simulink model "Prueba_PID"  (R2015b)
settings: Solver=ode45  StartTime=0  StopTime=1000  FixedStep=0.001  RelTol=1e-3
libraries: simulink_extras x20, simulink x6, aerolibtransform2 x4, aerolibutil x4, aerolibobsolete x2, aerolibasang x2
(part 1 of 3)
settings Model: Creator=David  LastModifiedBy=Juan
settings SolverCC: InitialStep=AUTO
settings DataIOCC: SaveCompleteFinalSimState=on  SaveFormat=Array  SaveState=on  ReturnWorkspaceOutputsName=simout
settings DebuggingCC: AlgebraicLoopMsg=none  UnderspecifiedInitializationDetection=Classic  MergeDetectMultiDrivingBlocksExec=none  StateNameClashWarn=warning
settings HardwareCC: ProdBitPerPointer=32  ProdLargestAtomicFloat=None  ProdIntDivRoundTo=Undefined  ProdEndianess=Unspecified  ProdWordSize=32  ProdHWDeviceType=32-bit Generic
settings GRTTargetCC: GeneratePreprocessorConditionals=Disable all
settings ConfigComp: CovModelRefEnable=Off

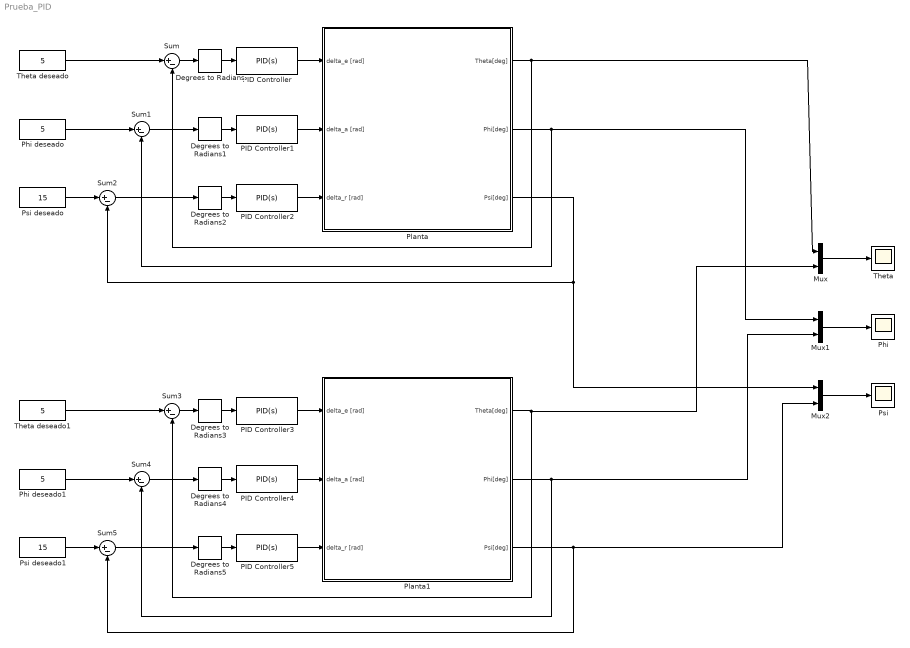
== system Prueba_PID ==
  Degrees to Radians{,1..5} (6 alike) : simulink_extras/Transformations/Degrees to Radians
  Mux : Mux  Inputs=2
  Mux1 : Mux  Inputs=2
  Mux2 : Mux  Inputs=2
  PID Controller : simulink/Continuous/PID Controller  Controller=PID  TimeDomain=Continuous-time  SampleTime=-1  IntegratorMethod=Forward Euler  FilterMethod=Forward Euler  Form=Parallel  UseFilter=on  ControllerParametersSource=internal  P=-1  I=-0.008  D=0.09  N=2  InitialConditionSource=internal  InitialConditionForIntegrator=0  InitialConditionForFilter=0  ExternalReset=none  LimitOutput=on  UpperSaturationLimit=0.062  LowerSaturationLimit=-0.062  LinearizeAsGain=on  AntiWindupMode=none  Kb=1  TrackingMode=off  Kt=1  PParamMin=[]  PParamMax=[]  IParamMin=[]  IParamMax=[]  DParamMin=[]  DParamMax=[]  NParamMin=[]  NParamMax=[]  KbParamMin=[]  KbParamMax=[]  KtParamMin=[]  KtParamMax=[]  POutMin=[]  POutMax=[]  IOutMin=[]  IOutMax=[]  DOutMin=[]  DOutMax=[]  NOutMin=[]  NOutMax=[]  KbOutMin=[]  KbOutMax=[]  KtOutMin=[]  KtOutMax=[]  IntegratorOutMin=[]  IntegratorOutMax=[]  FilterOutMin=[]  FilterOutMax=[]  SumOutMin=[]  SumOutMax=[]  SumI1OutMin=[]  SumI1OutMax=[]  SumI2OutMin=[]  SumI2OutMax=[]  SumI3OutMin=[]  SumI3OutMax=[]  SumDOutMin=[]  SumDOutMax=[]  SaturationOutMin=[]  SaturationOutMax=[]  IntegratorContinuousStateAttributes=''  IntegratorStateMustResolveToSignalObject=off  IntegratorRTWStateStorageClass=Auto  FilterContinuousStateAttributes=''  FilterStateMustResolveToSignalObject=off  FilterRTWStateStorageClass=Auto  DifferentiatorICPrevScaledInput=0  DifferentiatorOutMin=[]  DifferentiatorOutMax=[]
  PID Controller1 : simulink/Continuous/PID Controller  Controller=PID  TimeDomain=Continuous-time  SampleTime=-1  IntegratorMethod=Forward Euler  FilterMethod=Forward Euler  Form=Parallel  UseFilter=on  ControllerParametersSource=internal  P=0.09  I=0.001  D=2  N=2  InitialConditionSource=internal  InitialConditionForIntegrator=0  InitialConditionForFilter=0  ExternalReset=none  LimitOutput=on  UpperSaturationLimit=0.062  LowerSaturationLimit=-0.062  LinearizeAsGain=on  AntiWindupMode=none  Kb=1  TrackingMode=off  Kt=1  PParamMin=[]  PParamMax=[]  IParamMin=[]  IParamMax=[]  DParamMin=[]  DParamMax=[]  NParamMin=[]  NParamMax=[]  KbParamMin=[]  KbParamMax=[]  KtParamMin=[]  KtParamMax=[]  POutMin=[]  POutMax=[]  IOutMin=[]  IOutMax=[]  DOutMin=[]  DOutMax=[]  NOutMin=[]  NOutMax=[]  KbOutMin=[]  KbOutMax=[]  KtOutMin=[]  KtOutMax=[]  IntegratorOutMin=[]  IntegratorOutMax=[]  FilterOutMin=[]  FilterOutMax=[]  SumOutMin=[]  SumOutMax=[]  SumI1OutMin=[]  SumI1OutMax=[]  SumI2OutMin=[]  SumI2OutMax=[]  SumI3OutMin=[]  SumI3OutMax=[]  SumDOutMin=[]  SumDOutMax=[]  SaturationOutMin=[]  SaturationOutMax=[]  IntegratorContinuousStateAttributes=''  IntegratorStateMustResolveToSignalObject=off  IntegratorRTWStateStorageClass=Auto  FilterContinuousStateAttributes=''  FilterStateMustResolveToSignalObject=off  FilterRTWStateStorageClass=Auto  DifferentiatorICPrevScaledInput=0  DifferentiatorOutMin=[]  DifferentiatorOutMax=[]
  PID Controller2 : simulink/Continuous/PID Controller  Controller=PID  TimeDomain=Continuous-time  SampleTime=-1  IntegratorMethod=Forward Euler  FilterMethod=Forward Euler  Form=Parallel  UseFilter=on  ControllerParametersSource=internal  P=-0.5  I=-0.005  D=-0.01  N=2  InitialConditionSource=internal  InitialConditionForIntegrator=0  InitialConditionForFilter=0  ExternalReset=none  LimitOutput=on  UpperSaturationLimit=0.062  LowerSaturationLimit=-0.062  LinearizeAsGain=on  AntiWindupMode=none  Kb=1  TrackingMode=off  Kt=1  PParamMin=[]  PParamMax=[]  IParamMin=[]  IParamMax=[]  DParamMin=[]  DParamMax=[]  NParamMin=[]  NParamMax=[]  KbParamMin=[]  KbParamMax=[]  KtParamMin=[]  KtParamMax=[]  POutMin=[]  POutMax=[]  IOutMin=[]  IOutMax=[]  DOutMin=[]  DOutMax=[]  NOutMin=[]  NOutMax=[]  KbOutMin=[]  KbOutMax=[]  KtOutMin=[]  KtOutMax=[]  IntegratorOutMin=[]  IntegratorOutMax=[]  FilterOutMin=[]  FilterOutMax=[]  SumOutMin=[]  SumOutMax=[]  SumI1OutMin=[]  SumI1OutMax=[]  SumI2OutMin=[]  SumI2OutMax=[]  SumI3OutMin=[]  SumI3OutMax=[]  SumDOutMin=[]  SumDOutMax=[]  SaturationOutMin=[]  SaturationOutMax=[]  IntegratorContinuousStateAttributes=''  IntegratorStateMustResolveToSignalObject=off  IntegratorRTWStateStorageClass=Auto  FilterContinuousStateAttributes=''  FilterStateMustResolveToSignalObject=off  FilterRTWStateStorageClass=Auto  DifferentiatorICPrevScaledInput=0  DifferentiatorOutMin=[]  DifferentiatorOutMax=[]
  PID Controller3 : simulink/Continuous/PID Controller  Controller=PID  TimeDomain=Continuous-time  SampleTime=-1  IntegratorMethod=Forward Euler  FilterMethod=Forward Euler  Form=Parallel  UseFilter=on  ControllerParametersSource=internal  P=-1  I=-0.008  D=0.09  N=2  InitialConditionSource=internal  InitialConditionForIntegrator=0  InitialConditionForFilter=0  ExternalReset=none  LimitOutput=on  UpperSaturationLimit=0.062  LowerSaturationLimit=-0.062  LinearizeAsGain=on  AntiWindupMode=none  Kb=1  TrackingMode=off  Kt=1  PParamMin=[]  PParamMax=[]  IParamMin=[]  IParamMax=[]  DParamMin=[]  DParamMax=[]  NParamMin=[]  NParamMax=[]  KbParamMin=[]  KbParamMax=[]  KtParamMin=[]  KtParamMax=[]  POutMin=[]  POutMax=[]  IOutMin=[]  IOutMax=[]  DOutMin=[]  DOutMax=[]  NOutMin=[]  NOutMax=[]  KbOutMin=[]  KbOutMax=[]  KtOutMin=[]  KtOutMax=[]  IntegratorOutMin=[]  IntegratorOutMax=[]  FilterOutMin=[]  FilterOutMax=[]  SumOutMin=[]  SumOutMax=[]  SumI1OutMin=[]  SumI1OutMax=[]  SumI2OutMin=[]  SumI2OutMax=[]  SumI3OutMin=[]  SumI3OutMax=[]  SumDOutMin=[]  SumDOutMax=[]  SaturationOutMin=[]  SaturationOutMax=[]  IntegratorContinuousStateAttributes=''  IntegratorStateMustResolveToSignalObject=off  IntegratorRTWStateStorageClass=Auto  FilterContinuousStateAttributes=''  FilterStateMustResolveToSignalObject=off  FilterRTWStateStorageClass=Auto  DifferentiatorICPrevScaledInput=0  DifferentiatorOutMin=[]  DifferentiatorOutMax=[]
  PID Controller4 : simulink/Continuous/PID Controller  Controller=PID  TimeDomain=Continuous-time  SampleTime=-1  IntegratorMethod=Forward Euler  FilterMethod=Forward Euler  Form=Parallel  UseFilter=on  ControllerParametersSource=internal  P=0.09  I=0.001  D=2  N=2  InitialConditionSource=internal  InitialConditionForIntegrator=0  InitialConditionForFilter=0  ExternalReset=none  LimitOutput=on  UpperSaturationLimit=0.062  LowerSaturationLimit=-0.062  LinearizeAsGain=on  AntiWindupMode=none  Kb=1  TrackingMode=off  Kt=1  PParamMin=[]  PParamMax=[]  IParamMin=[]  IParamMax=[]  DParamMin=[]  DParamMax=[]  NParamMin=[]  NParamMax=[]  KbParamMin=[]  KbParamMax=[]  KtParamMin=[]  KtParamMax=[]  POutMin=[]  POutMax=[]  IOutMin=[]  IOutMax=[]  DOutMin=[]  DOutMax=[]  NOutMin=[]  NOutMax=[]  KbOutMin=[]  KbOutMax=[]  KtOutMin=[]  KtOutMax=[]  IntegratorOutMin=[]  IntegratorOutMax=[]  FilterOutMin=[]  FilterOutMax=[]  SumOutMin=[]  SumOutMax=[]  SumI1OutMin=[]  SumI1OutMax=[]  SumI2OutMin=[]  SumI2OutMax=[]  SumI3OutMin=[]  SumI3OutMax=[]  SumDOutMin=[]  SumDOutMax=[]  SaturationOutMin=[]  SaturationOutMax=[]  IntegratorContinuousStateAttributes=''  IntegratorStateMustResolveToSignalObject=off  IntegratorRTWStateStorageClass=Auto  FilterContinuousStateAttributes=''  FilterStateMustResolveToSignalObject=off  FilterRTWStateStorageClass=Auto  DifferentiatorICPrevScaledInput=0  DifferentiatorOutMin=[]  DifferentiatorOutMax=[]
  PID Controller5 : simulink/Continuous/PID Controller  Controller=PID  TimeDomain=Continuous-time  SampleTime=-1  IntegratorMethod=Forward Euler  FilterMethod=Forward Euler  Form=Parallel  UseFilter=on  ControllerParametersSource=internal  P=-0.5  I=-0.005  D=-0.01  N=2  InitialConditionSource=internal  InitialConditionForIntegrator=0  InitialConditionForFilter=0  ExternalReset=none  LimitOutput=on  UpperSaturationLimit=0.062  LowerSaturationLimit=-0.062  LinearizeAsGain=on  AntiWindupMode=none  Kb=1  TrackingMode=off  Kt=1  PParamMin=[]  PParamMax=[]  IParamMin=[]  IParamMax=[]  DParamMin=[]  DParamMax=[]  NParamMin=[]  NParamMax=[]  KbParamMin=[]  KbParamMax=[]  KtParamMin=[]  KtParamMax=[]  POutMin=[]  POutMax=[]  IOutMin=[]  IOutMax=[]  DOutMin=[]  DOutMax=[]  NOutMin=[]  NOutMax=[]  KbOutMin=[]  KbOutMax=[]  KtOutMin=[]  KtOutMax=[]  IntegratorOutMin=[]  IntegratorOutMax=[]  FilterOutMin=[]  FilterOutMax=[]  SumOutMin=[]  SumOutMax=[]  SumI1OutMin=[]  SumI1OutMax=[]  SumI2OutMin=[]  SumI2OutMax=[]  SumI3OutMin=[]  SumI3OutMax=[]  SumDOutMin=[]  SumDOutMax=[]  SaturationOutMin=[]  SaturationOutMax=[]  IntegratorContinuousStateAttributes=''  IntegratorStateMustResolveToSignalObject=off  IntegratorRTWStateStorageClass=Auto  FilterContinuousStateAttributes=''  FilterStateMustResolveToSignalObject=off  FilterRTWStateStorageClass=Auto  DifferentiatorICPrevScaledInput=0  DifferentiatorOutMin=[]  DifferentiatorOutMax=[]
  "Phi " : Scope
  Phi deseado : Constant  Value=5
  Phi deseado1 : Constant  Value=5
  Planta : Subsystem
  Planta1 : Subsystem
  Psi : Scope
  Psi deseado : Constant  Value=15
  Psi deseado1 : Constant  Value=15
  Sum{,1..5} (6 alike) : Sum  Inputs=|+-
  Theta : Scope
  Theta deseado : Constant  Value=5
  Theta deseado1 : Constant  Value=5
  wires:
  Theta deseado/1 -> Sum/1
  PID Controller/1 -> Planta/1(delta_e [rad])
  Planta/1(Theta[deg]) -> Sum/2, Mux/1
  Planta/3(Psi[deg]) -> Mux2/1, Sum2/2
  Planta/2(Phi[deg]) -> Sum1/2, Mux1/1
  PID Controller1/1 -> Planta/2(delta_a [rad])
  PID Controller2/1 -> Planta/3(delta_r [rad])
  Phi deseado/1 -> Sum1/1
  Degrees to Radians/1 -> PID Controller/1
  Sum/1 -> Degrees to Radians/1
  Sum1/1 -> Degrees to Radians1/1
  Degrees to Radians1/1 -> PID Controller1/1
  Degrees to Radians2/1 -> PID Controller2/1
  Psi deseado/1 -> Sum2/1
  Sum2/1 -> Degrees to Radians2/1
  Theta deseado1/1 -> Sum3/1
  PID Controller3/1 -> Planta1/1(delta_e [rad])
  Planta1/1(Theta[deg]) -> Mux/2, Sum3/2
  Planta1/3(Psi[deg]) -> Sum5/2, Mux2/2
  Planta1/2(Phi[deg]) -> Mux1/2, Sum4/2
  PID Controller4/1 -> Planta1/2(delta_a [rad])
  PID Controller5/1 -> Planta1/3(delta_r [rad])
  Phi deseado1/1 -> Sum4/1
  Degrees to Radians3/1 -> PID Controller3/1
  Sum3/1 -> Degrees to Radians3/1
  Sum4/1 -> Degrees to Radians4/1
  Degrees to Radians4/1 -> PID Controller4/1
  Degrees to Radians5/1 -> PID Controller5/1
  Psi deseado1/1 -> Sum5/1
  Sum5/1 -> Degrees to Radians5/1
  Mux/1 -> Theta/1
  Mux1/1 -> "Phi "/1
  Mux2/1 -> Psi/1

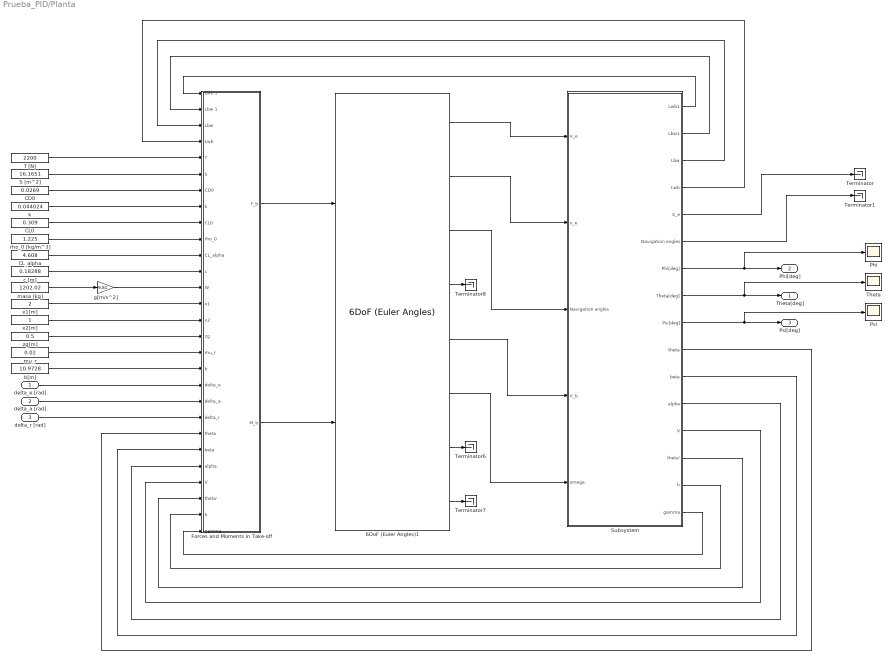
== system Prueba_PID/Planta ==
  delta_e [rad] : Inport
  delta_a [rad] : Inport  Port=2
  delta_r [rad] : Inport  Port=3
  6DoF (Euler Angles)1 : aerolibobsolete/6DoF (Euler Angles)  units=Metric (MKS)  mtype=Fixed  rep=Euler Angles  xme_0=[0 0 0]  Vm_0=[0.01 0 0]  eul_0=[0 0.035 0]  pm_0=[0 0 0]  mass_0=Mass  mass_e=0.5  mass_f=2.0  inertia=Inertia  inertia_e=eye(3)  inertia_f=2*eye(3)  k_quat=1.0
  CD0 : Constant  Value=0.0269
  CL0 : Constant  Value=0.309
  "CL_alpha " : Constant  Value=4.608
  Forces and Moments in Take-off : Subsystem
  Phi : Scope
  Psi : Scope
  S [m^2] : Constant  Value=16.1651
  Subsystem : Subsystem
  T [N] : Constant  Value=2200
  Terminator{,1,6..8} (5 alike) : Terminator
  Theta : Scope
  b[m] : Constant  Value=10.9728
  c [m] : Constant  Value=0.18288
  g[m/s^2] : Gain  Gain=9.81
  k : Constant  Value=0.044024
  "masa [kg] " : Constant  Value=1202.02
  "mu_r " : Constant  Value=0.02
  rho_0 [kg/m^3] : Constant  Value=1.225
  x1[m] : Constant  Value=2
  x2[m] : Constant
  zg[m] : Constant  Value=0.5
  Theta[deg] : Outport
  Phi[deg] : Outport  Port=2
  Psi[deg] : Outport  Port=3
  wires:
  T [N]/1 -> Forces and Moments in Take-off/5(T)
  S [m^2]/1 -> Forces and Moments in Take-off/6(S)
  CD0/1 -> Forces and Moments in Take-off/7(CD0)
  "masa [kg] "/1 -> g[m/s^2]/1
  k/1 -> Forces and Moments in Take-off/8(k)
  zg[m]/1 -> Forces and Moments in Take-off/16(zg)
  CL0/1 -> Forces and Moments in Take-off/9(CL0)
  rho_0 [kg/m^3]/1 -> Forces and Moments in Take-off/10(rho_0)
  "CL_alpha "/1 -> Forces and Moments in Take-off/11(CL_alpha)
  c [m]/1 -> Forces and Moments in Take-off/12(c)
  g[m/s^2]/1 -> Forces and Moments in Take-off/13(W)
  x1[m]/1 -> Forces and Moments in Take-off/14(x1)
  x2[m]/1 -> Forces and Moments in Take-off/15(x2)
  "mu_r "/1 -> Forces and Moments in Take-off/17(mu_r)
  delta_e [rad]/1 -> Forces and Moments in Take-off/19(delta_e)
  delta_a [rad]/1 -> Forces and Moments in Take-off/20(delta_a)
  delta_r [rad]/1 -> Forces and Moments in Take-off/21(delta_r)
  b[m]/1 -> Forces and Moments in Take-off/18(b)
  6DoF (Euler Angles)1/7 -> Terminator6/1
  6DoF (Euler Angles)1/8 -> Terminator7/1
  6DoF (Euler Angles)1/4 -> Terminator8/1
  Forces and Moments in Take-off/1(F_b) -> 6DoF (Euler Angles)1/1
  Forces and Moments in Take-off/2(M_b) -> 6DoF (Euler Angles)1/2
  6DoF (Euler Angles)1/1 -> Subsystem/1(V_e)
  6DoF (Euler Angles)1/2 -> Subsystem/2(x_e)
  6DoF (Euler Angles)1/5 -> Subsystem/4(V_b)
  6DoF (Euler Angles)1/6 -> Subsystem/5(omega)
  Subsystem/1(Lwb1) -> Forces and Moments in Take-off/1(Lwb 1)
  Subsystem/2(Lbw1) -> Forces and Moments in Take-off/2(Lbw 1)
  Subsystem/3("Lbw ") -> Forces and Moments in Take-off/3(Lbw)
  Subsystem/4(Lwb) -> Forces and Moments in Take-off/4(Lwb)
  Subsystem/8(Theta[deg]) -> Theta/1, Theta[deg]/1
  Subsystem/10(theta) -> Forces and Moments in Take-off/22(theta)
  Subsystem/11(beta) -> Forces and Moments in Take-off/23(beta)
  Subsystem/12(alpha) -> Forces and Moments in Take-off/24("alpha ")
  Subsystem/13(V) -> Forces and Moments in Take-off/25(V)
  Subsystem/14(theta') -> Forces and Moments in Take-off/26(theta')
  Subsystem/15(h) -> Forces and Moments in Take-off/27(h)
  Subsystem/16(gamma) -> Forces and Moments in Take-off/28(gamma)
  Subsystem/9(Psi[deg]) -> Psi/1, Psi[deg]/1
  Subsystem/7(Phi[deg]) -> Phi/1, Phi[deg]/1
  6DoF (Euler Angles)1/3 -> Subsystem/3(Navigation angles)
  Subsystem/5(X_e) -> Terminator/1
  Subsystem/6("Navigation angles ") -> Terminator1/1

== system Prueba_PID/Planta1 ==
  delta_e [rad] : Inport
  delta_a [rad] : Inport  Port=2
  delta_r [rad] : Inport  Port=3
  6DoF (Euler Angles)1 : aerolibobsolete/6DoF (Euler Angles)  units=Metric (MKS)  mtype=Fixed  rep=Euler Angles  xme_0=[0 0 0]  Vm_0=[0.01 0 0]  eul_0=[0 0.035 0]  pm_0=[0 0 0]  mass_0=Mass  mass_e=0.5  mass_f=2.0  inertia=Inertia  inertia_e=eye(3)  inertia_f=2*eye(3)  k_quat=1.0
  CD0 : Constant  Value=0.0269
  CL0 : Constant  Value=0.309
  "CL_alpha " : Constant  Value=4.608
  Forces and Moments in Take-off : Subsystem
  Phi : Scope
  Psi : Scope
  S [m^2] : Constant  Value=16.1651
  Subsystem : Subsystem
  T [N] : Constant  Value=2200
  Terminator{,1,6..8} (5 alike) : Terminator
  Theta : Scope
  b[m] : Constant  Value=10.9728
  c [m] : Constant  Value=0.18288
  g[m/s^2] : Gain  Gain=9.81
  k : Constant  Value=0.044024
  "masa [kg] " : Constant  Value=1202.02
  "mu_r " : Constant  Value=0.02
  rho_0 [kg/m^3] : Constant  Value=1.225
  x1[m] : Constant  Value=2
  x2[m] : Constant
  zg[m] : Constant  Value=0.5
  Theta[deg] : Outport
  Phi[deg] : Outport  Port=2
  Psi[deg] : Outport  Port=3
  wires:
  T [N]/1 -> Forces and Moments in Take-off/5(T)
  S [m^2]/1 -> Forces and Moments in Take-off/6(S)
  CD0/1 -> Forces and Moments in Take-off/7(CD0)
  "masa [kg] "/1 -> g[m/s^2]/1
  k/1 -> Forces and Moments in Take-off/8(k)
  zg[m]/1 -> Forces and Moments in Take-off/16(zg)
  CL0/1 -> Forces and Moments in Take-off/9(CL0)
  rho_0 [kg/m^3]/1 -> Forces and Moments in Take-off/10(rho_0)
  "CL_alpha "/1 -> Forces and Moments in Take-off/11(CL_alpha)
  c [m]/1 -> Forces and Moments in Take-off/12(c)
  g[m/s^2]/1 -> Forces and Moments in Take-off/13(W)
  x1[m]/1 -> Forces and Moments in Take-off/14(x1)
  x2[m]/1 -> Forces and Moments in Take-off/15(x2)
  "mu_r "/1 -> Forces and Moments in Take-off/17(mu_r)
  delta_e [rad]/1 -> Forces and Moments in Take-off/19(delta_e)
  delta_a [rad]/1 -> Forces and Moments in Take-off/20(delta_a)
  delta_r [rad]/1 -> Forces and Moments in Take-off/21(delta_r)
  b[m]/1 -> Forces and Moments in Take-off/18(b)
  6DoF (Euler Angles)1/7 -> Terminator6/1
  6DoF (Euler Angles)1/8 -> Terminator7/1
  6DoF (Euler Angles)1/4 -> Terminator8/1
  Forces and Moments in Take-off/1(F_b) -> 6DoF (Euler Angles)1/1
  Forces and Moments in Take-off/2(M_b) -> 6DoF (Euler Angles)1/2
  6DoF (Euler Angles)1/1 -> Subsystem/1(V_e)
  6DoF (Euler Angles)1/2 -> Subsystem/2(x_e)
  6DoF (Euler Angles)1/5 -> Subsystem/4(V_b)
  6DoF (Euler Angles)1/6 -> Subsystem/5(omega)
  Subsystem/1(Lwb1) -> Forces and Moments in Take-off/1(Lwb 1)
  Subsystem/2(Lbw1) -> Forces and Moments in Take-off/2(Lbw 1)
  Subsystem/3("Lbw ") -> Forces and Moments in Take-off/3(Lbw)
  Subsystem/4(Lwb) -> Forces and Moments in Take-off/4(Lwb)
  Subsystem/8(Theta[deg]) -> Theta/1, Theta[deg]/1
  Subsystem/10(theta) -> Forces and Moments in Take-off/22(theta)
  Subsystem/11(beta) -> Forces and Moments in Take-off/23(beta)
  Subsystem/12(alpha) -> Forces and Moments in Take-off/24("alpha ")
  Subsystem/13(V) -> Forces and Moments in Take-off/25(V)
  Subsystem/14(theta') -> Forces and Moments in Take-off/26(theta')
  Subsystem/15(h) -> Forces and Moments in Take-off/27(h)
  Subsystem/16(gamma) -> Forces and Moments in Take-off/28(gamma)
  Subsystem/9(Psi[deg]) -> Psi/1, Psi[deg]/1
  Subsystem/7(Phi[deg]) -> Phi/1, Phi[deg]/1
  6DoF (Euler Angles)1/3 -> Subsystem/3(Navigation angles)
  Subsystem/5(X_e) -> Terminator/1
  Subsystem/6("Navigation angles ") -> Terminator1/1

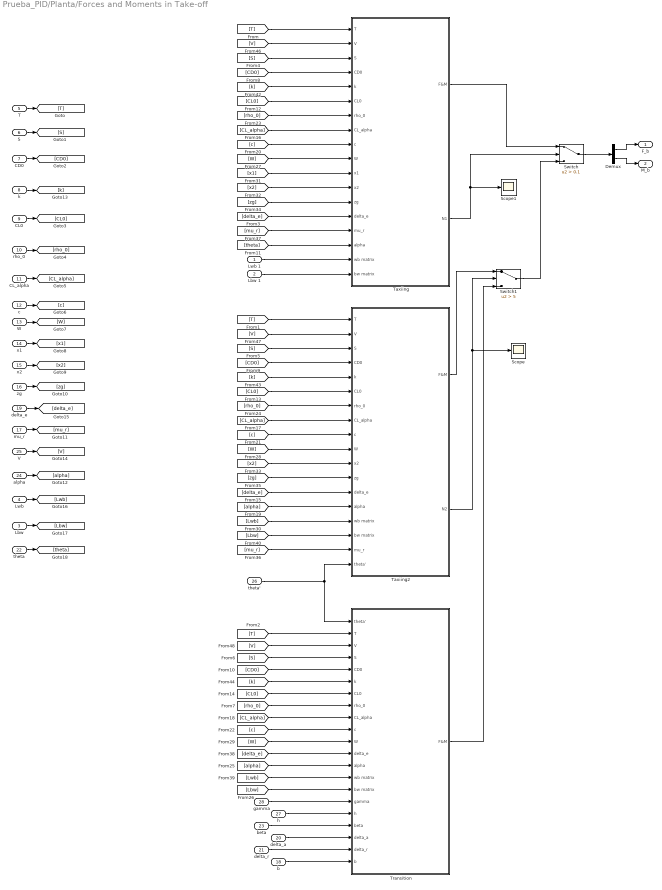
== system Prueba_PID/Planta/Forces and Moments in Take-off ==
  Lwb 1 : Inport
  Lbw 1 : Inport  Port=2
  Lbw : Inport  Port=3
  Lwb : Inport  Port=4
  T : Inport  Port=5
  S : Inport  Port=6
  CD0 : Inport  Port=7
  k : Inport  Port=8
  CL0 : Inport  Port=9
  rho_0 : Inport  Port=10
  CL_alpha : Inport  Port=11
  c : Inport  Port=12
  W : Inport  Port=13
  x1 : Inport  Port=14
  x2 : Inport  Port=15
  zg : Inport  Port=16
  mu_r : Inport  Port=17
  b : Inport  Port=18
  delta_e : Inport  Port=19
  delta_a : Inport  Port=20
  delta_r : Inport  Port=21
  theta : Inport  Port=22
  beta : Inport  Port=23
  "alpha " : Inport  Port=24
  V : Inport  Port=25
  theta' : Inport  Port=26
  h : Inport  Port=27
  gamma : Inport  Port=28
  Demux : Demux  Outputs=2
  Scope : Scope
  Scope1 : Scope
  Switch : Switch  Criteria=u2 > Threshold  Threshold=0.1
  Switch1 : Switch  Criteria=u2 > Threshold  Threshold=5  ZeroCross=off
  Taxiing : Subsystem
  Taxiing2 : Subsystem
  Transition : Subsystem
  F_b : Outport
  M_b : Outport  Port=2
  wires:
  Taxiing/1(F&M) -> Switch/1
  theta'/1 -> Taxiing2/18(theta'), Transition/1(theta')
  Switch1/1 -> Switch/3
  Switch/1 -> Demux/1
  Taxiing2/1(F&M) -> Switch1/1
  Demux/2 -> M_b/1
  Taxiing2/2(N2) -> Switch1/2, Scope/1
  Demux/1 -> F_b/1
  T/1 -> [T]
  [T] -> Taxiing2/1(T)
  [T] -> Transition/2(T)
  S/1 -> [S]
  CD0/1 -> [CD0]
  CL0/1 -> [CL0]
  rho_0/1 -> [rho_0]
  CL_alpha/1 -> [CL_alpha]
  c/1 -> [c]
  W/1 -> [W]
  x1/1 -> [x1]
  x2/1 -> [x2]
  zg/1 -> [zg]
  [S] -> Taxiing2/3(S)
  [S] -> Transition/4(S)
  [CD0] -> Taxiing2/4(CD0)
  [CD0] -> Transition/5(CD0)
  [CL0] -> Taxiing2/6(CL0)
  [CL0] -> Transition/7(CL0)
  [CL_alpha] -> Taxiing2/8(CL_alpha)
  [CL_alpha] -> Transition/9(CL_alpha)
  [c] -> Taxiing2/9(c)
  [c] -> Transition/10(c)
  [rho_0] -> Taxiing2/7(rho_0)
  [rho_0] -> Transition/8(rho_0)
  [W] -> Taxiing2/10(W)
  [W] -> Transition/11(W)
  [x2] -> Taxiing2/11(x2)
  [zg] -> Taxiing2/12(zg)
  mu_r/1 -> [mu_r]
  [mu_r] -> Taxiing2/17(mu_r)
  delta_e/1 -> [delta_e]
  [delta_e] -> Transition/12(delta_e)
  [delta_e] -> Taxiing2/13(delta_e)
  k/1 -> [k]
  [k] -> Taxiing2/5(k)
  [k] -> Transition/6(k)
  V/1 -> [V]
  [V] -> Taxiing2/2(V)
  [V] -> Transition/3(V)
  Transition/1(F&M) -> Switch1/3
  Taxiing/2(N1) -> Switch/2, Scope1/1
  h/1 -> Transition/17(h)
  beta/1 -> Transition/18(beta)
  gamma/1 -> Transition/16(gamma)
  delta_a/1 -> Transition/19(delta_a)
  delta_r/1 -> Transition/20(delta_r)
  b/1 -> Transition/21(b)
  "alpha "/1 -> [alpha]
  [alpha] -> Taxiing2/14(alpha)
  [alpha] -> Transition/13(alpha)
  [Lbw] -> Transition/15(bw matrix)
  [Lwb] -> Taxiing2/15(wb matrix)
  [Lwb] -> Transition/14(wb matrix)
  [Lbw] -> Taxiing2/16(bw matrix)
  Lwb/1 -> [Lwb]
  Lbw/1 -> [Lbw]
  [T] -> Taxiing/1(T)
  Lbw 1/1 -> Taxiing/18(bw matrix)
  Lwb 1/1 -> Taxiing/17(wb matrix)
  [theta] -> Taxiing/16(alpha)
  [mu_r] -> Taxiing/15(mu_r)
  [delta_e] -> Taxiing/14(delta_e)
  [zg] -> Taxiing/13(zg)
  [x2] -> Taxiing/12(x2)
  [x1] -> Taxiing/11(x1)
  [W] -> Taxiing/10(W)
  [c] -> Taxiing/9(c)
  [CL_alpha] -> Taxiing/8(CL_alpha)
  [rho_0] -> Taxiing/7(rho_0)
  [CL0] -> Taxiing/6(CL0)
  [k] -> Taxiing/5(k)
  [CD0] -> Taxiing/4(CD0)
  [S] -> Taxiing/3(S)
  [V] -> Taxiing/2(V)
  theta/1 -> [theta]

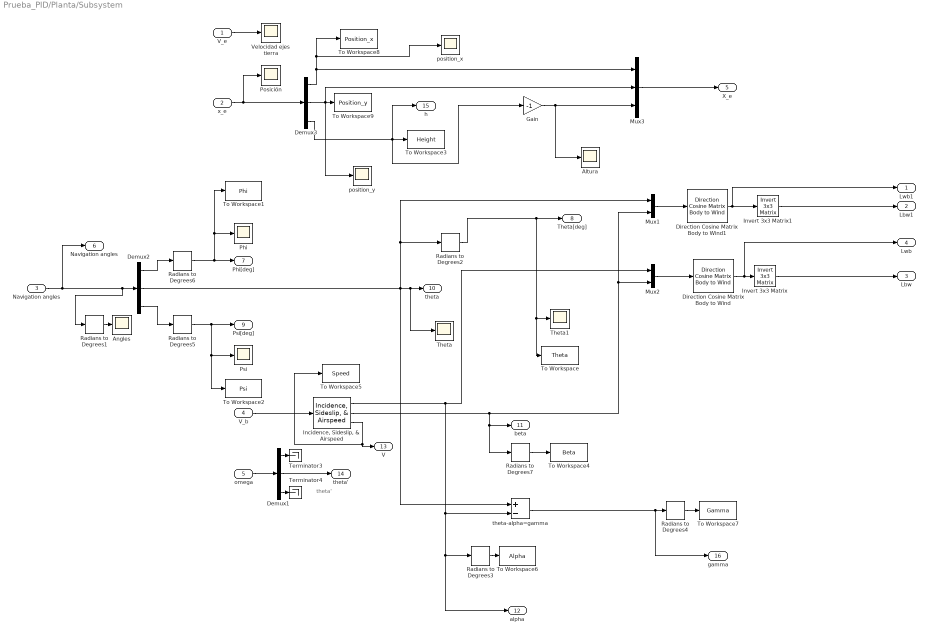
== system Prueba_PID/Planta/Subsystem ==
  note: theta'
  V_e : Inport
  x_e : Inport  Port=2
  Navigation angles : Inport  Port=3
  V_b : Inport  Port=4
  omega : Inport  Port=5
  Altura : Scope
  Angles : Scope
  Demux1 : Demux  Outputs=3
  Demux2 : Demux  Outputs=3
  Demux3 : Demux  Outputs=3
  Direction Cosine Matrix Body to Wind : aerolibtransform2/Direction Cosine Matrix Body to Wind
  Direction Cosine Matrix Body to Wind1 : aerolibtransform2/Direction Cosine Matrix Body to Wind
  Gain : Gain  Gain=-1
  "Incidence, Sideslip, & Airspeed" : aerolibasang/Incidence, Sideslip, & Airspeed
  Invert 3x3 Matrix : aerolibutil/Invert  3x3 Matrix
  Invert 3x3 Matrix1 : aerolibutil/Invert  3x3 Matrix
  Mux1 : Mux  Inputs=2
  Mux2 : Mux  Inputs=2
  Mux3 : Mux  Inputs=3
  Phi : Scope
  Posición : Scope
  Psi : Scope
  Radians to Degrees{1..7} (7 alike) : simulink_extras/Transformations/Radians to Degrees
  Terminator3 : Terminator
  Terminator4 : Terminator
  Theta : Scope
  Theta1 : Scope
  To Workspace : ToWorkspace  VariableName=Theta  SampleTime=-1
  To Workspace1 : ToWorkspace  VariableName=Phi  SampleTime=-1
  To Workspace2 : ToWorkspace  VariableName=Psi  SampleTime=-1
  To Workspace3 : ToWorkspace  VariableName=Height  SampleTime=-1
  To Workspace4 : ToWorkspace  VariableName=Beta  SampleTime=-1
  To Workspace5 : ToWorkspace  VariableName=Speed  SampleTime=-1
  To Workspace6 : ToWorkspace  VariableName=Alpha  SampleTime=-1
  To Workspace7 : ToWorkspace  VariableName=Gamma  SampleTime=-1
  To Workspace8 : ToWorkspace  VariableName=Position_x  SampleTime=-1
  To Workspace9 : ToWorkspace  VariableName=Position_y  SampleTime=-1
  "Velocidad ejes tierra " : Scope
  position_x : Scope
  position_y : Scope
  theta-alpha=gamma : Sum  Inputs=+-
  Lwb1 : Outport
  Lbw1 : Outport  Port=2
  "Lbw " : Outport  Port=3
  Lwb : Outport  Port=4
  X_e : Outport  Port=5
  "Navigation angles " : Outport  Port=6
  Phi[deg] : Outport  Port=7
  Theta[deg] : Outport  Port=8
  Psi[deg] : Outport  Port=9
  theta : Outport  Port=10
  beta : Outport  Port=11
  alpha : Outport  Port=12
  V : Outport  Port=13
  theta' : Outport  Port=14
  h : Outport  Port=15
  gamma : Outport  Port=16
  wires:
  Direction Cosine Matrix Body to Wind/1 -> Lwb/1, Invert 3x3 Matrix/1
  Radians to Degrees3/1 -> To Workspace6/1
  theta-alpha=gamma/1 -> gamma/1, Radians to Degrees4/1
  Invert 3x3 Matrix/1 -> "Lbw "/1
  Mux1/1 -> Direction Cosine Matrix Body to Wind1/1
  Demux3/3 -> Gain/1, h/1, To Workspace3/1
  V_e/1 -> "Velocidad ejes tierra "/1
  omega/1 -> Demux1/1
  "Incidence, Sideslip, & Airspeed"/2 -> beta/1, Radians to Degrees7/1, Mux2/2, Mux1/2
  V_b/1 -> "Incidence, Sideslip, & Airspeed"/1
  x_e/1 -> Demux3/1, Posición/1
  Mux2/1 -> Direction Cosine Matrix Body to Wind/1
  Direction Cosine Matrix Body to Wind1/1 -> Lwb1/1, Invert 3x3 Matrix1/1
  "Incidence, Sideslip, & Airspeed"/1 -> Mux2/1, alpha/1, Radians to Degrees3/1, theta-alpha=gamma/2
  Radians to Degrees2/1 -> To Workspace/1, Theta1/1, Theta[deg]/1
  Demux1/3 -> Terminator4/1
  Demux1/2 -> theta'/1
  Invert 3x3 Matrix1/1 -> Lbw1/1
  Demux1/1 -> Terminator3/1
  Demux2/1 -> Radians to Degrees6/1
  Demux3/2 -> position_y/1, Mux3/2, To Workspace9/1
  Radians to Degrees1/1 -> Angles/1
  Demux3/1 -> Mux3/1, position_x/1, To Workspace8/1
  Demux2/2 -> theta-alpha=gamma/1, Theta/1, theta/1, Mux1/1, Radians to Degrees2/1
  Radians to Degrees4/1 -> To Workspace7/1
  "Incidence, Sideslip, & Airspeed"/3 -> V/1, To Workspace5/1
  Demux2/3 -> Radians to Degrees5/1
  Radians to Degrees5/1 -> To Workspace2/1, Psi/1, Psi[deg]/1
  Radians to Degrees6/1 -> To Workspace1/1, Phi/1, Phi[deg]/1
  Radians to Degrees7/1 -> To Workspace4/1
  Mux3/1 -> X_e/1
  Gain/1 -> Altura/1, Mux3/3
  Navigation angles/1 -> "Navigation angles "/1, Radians to Degrees1/1, Demux2/1

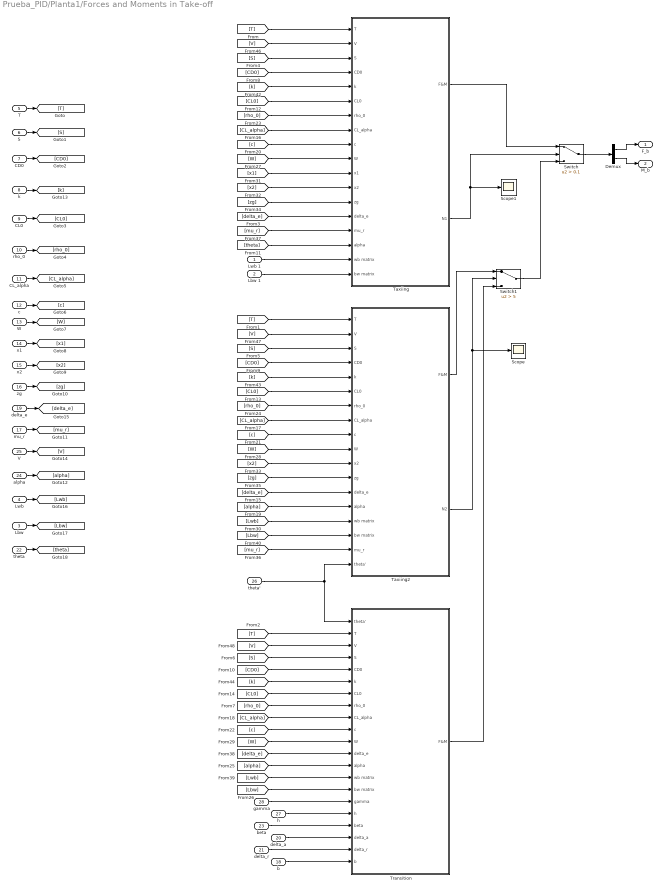
== system Prueba_PID/Planta1/Forces and Moments in Take-off ==
  Lwb 1 : Inport
  Lbw 1 : Inport  Port=2
  Lbw : Inport  Port=3
  Lwb : Inport  Port=4
  T : Inport  Port=5
  S : Inport  Port=6
  CD0 : Inport  Port=7
  k : Inport  Port=8
  CL0 : Inport  Port=9
  rho_0 : Inport  Port=10
  CL_alpha : Inport  Port=11
  c : Inport  Port=12
  W : Inport  Port=13
  x1 : Inport  Port=14
  x2 : Inport  Port=15
  zg : Inport  Port=16
  mu_r : Inport  Port=17
  b : Inport  Port=18
  delta_e : Inport  Port=19
  delta_a : Inport  Port=20
  delta_r : Inport  Port=21
  theta : Inport  Port=22
  beta : Inport  Port=23
  "alpha " : Inport  Port=24
  V : Inport  Port=25
  theta' : Inport  Port=26
  h : Inport  Port=27
  gamma : Inport  Port=28
  Demux : Demux  Outputs=2
  Scope : Scope
  Scope1 : Scope
  Switch : Switch  Criteria=u2 > Threshold  Threshold=0.1
  Switch1 : Switch  Criteria=u2 > Threshold  Threshold=5  ZeroCross=off
  Taxiing : Subsystem
  Taxiing2 : Subsystem
  Transition : Subsystem
  F_b : Outport
  M_b : Outport  Port=2
  wires:
  Taxiing/1(F&M) -> Switch/1
  theta'/1 -> Taxiing2/18(theta'), Transition/1(theta')
  Switch1/1 -> Switch/3
  Switch/1 -> Demux/1
  Taxiing2/1(F&M) -> Switch1/1
  Demux/2 -> M_b/1
  Taxiing2/2(N2) -> Switch1/2, Scope/1
  Demux/1 -> F_b/1
  T/1 -> [T]
  [T] -> Taxiing2/1(T)
  [T] -> Transition/2(T)
  S/1 -> [S]
  CD0/1 -> [CD0]
  CL0/1 -> [CL0]
  rho_0/1 -> [rho_0]
  CL_alpha/1 -> [CL_alpha]
  c/1 -> [c]
  W/1 -> [W]
  x1/1 -> [x1]
  x2/1 -> [x2]
  zg/1 -> [zg]
  [S] -> Taxiing2/3(S)
  [S] -> Transition/4(S)
  [CD0] -> Taxiing2/4(CD0)
  [CD0] -> Transition/5(CD0)
  [CL0] -> Taxiing2/6(CL0)
  [CL0] -> Transition/7(CL0)
  [CL_alpha] -> Taxiing2/8(CL_alpha)
  [CL_alpha] -> Transition/9(CL_alpha)
  [c] -> Taxiing2/9(c)
  [c] -> Transition/10(c)
  [rho_0] -> Taxiing2/7(rho_0)
  [rho_0] -> Transition/8(rho_0)
  [W] -> Taxiing2/10(W)
  [W] -> Transition/11(W)
  [x2] -> Taxiing2/11(x2)
  [zg] -> Taxiing2/12(zg)
  mu_r/1 -> [mu_r]
  [mu_r] -> Taxiing2/17(mu_r)
  delta_e/1 -> [delta_e]
  [delta_e] -> Transition/12(delta_e)
  [delta_e] -> Taxiing2/13(delta_e)
  k/1 -> [k]
  [k] -> Taxiing2/5(k)
  [k] -> Transition/6(k)
  V/1 -> [V]
  [V] -> Taxiing2/2(V)
  [V] -> Transition/3(V)
  Transition/1(F&M) -> Switch1/3
  Taxiing/2(N1) -> Switch/2, Scope1/1
  h/1 -> Transition/17(h)
  beta/1 -> Transition/18(beta)
  gamma/1 -> Transition/16(gamma)
  delta_a/1 -> Transition/19(delta_a)
  delta_r/1 -> Transition/20(delta_r)
  b/1 -> Transition/21(b)
  "alpha "/1 -> [alpha]
  [alpha] -> Taxiing2/14(alpha)
  [alpha] -> Transition/13(alpha)
  [Lbw] -> Transition/15(bw matrix)
  [Lwb] -> Taxiing2/15(wb matrix)
  [Lwb] -> Transition/14(wb matrix)
  [Lbw] -> Taxiing2/16(bw matrix)
  Lwb/1 -> [Lwb]
  Lbw/1 -> [Lbw]
  [T] -> Taxiing/1(T)
  Lbw 1/1 -> Taxiing/18(bw matrix)
  Lwb 1/1 -> Taxiing/17(wb matrix)
  [theta] -> Taxiing/16(alpha)
  [mu_r] -> Taxiing/15(mu_r)
  [delta_e] -> Taxiing/14(delta_e)
  [zg] -> Taxiing/13(zg)
  [x2] -> Taxiing/12(x2)
  [x1] -> Taxiing/11(x1)
  [W] -> Taxiing/10(W)
  [c] -> Taxiing/9(c)
  [CL_alpha] -> Taxiing/8(CL_alpha)
  [rho_0] -> Taxiing/7(rho_0)
  [CL0] -> Taxiing/6(CL0)
  [k] -> Taxiing/5(k)
  [CD0] -> Taxiing/4(CD0)
  [S] -> Taxiing/3(S)
  [V] -> Taxiing/2(V)
  theta/1 -> [theta]

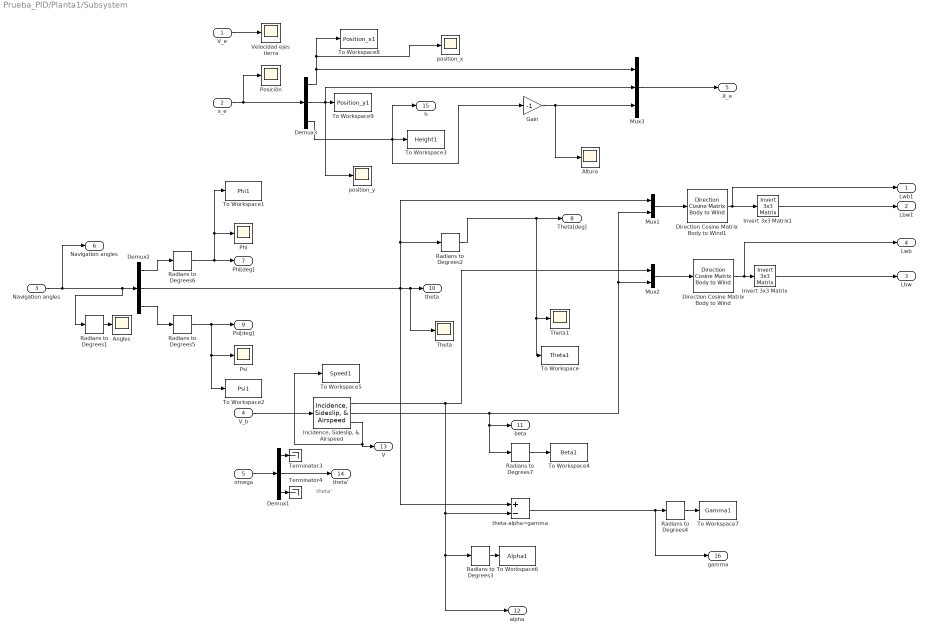
== system Prueba_PID/Planta1/Subsystem ==
  note: theta'
  V_e : Inport
  x_e : Inport  Port=2
  Navigation angles : Inport  Port=3
  V_b : Inport  Port=4
  omega : Inport  Port=5
  Altura : Scope
  Angles : Scope
  Demux1 : Demux  Outputs=3
  Demux2 : Demux  Outputs=3
  Demux3 : Demux  Outputs=3
  Direction Cosine Matrix Body to Wind : aerolibtransform2/Direction Cosine Matrix Body to Wind
  Direction Cosine Matrix Body to Wind1 : aerolibtransform2/Direction Cosine Matrix Body to Wind
  Gain : Gain  Gain=-1
  "Incidence, Sideslip, & Airspeed" : aerolibasang/Incidence, Sideslip, & Airspeed
  Invert 3x3 Matrix : aerolibutil/Invert  3x3 Matrix
  Invert 3x3 Matrix1 : aerolibutil/Invert  3x3 Matrix
  Mux1 : Mux  Inputs=2
  Mux2 : Mux  Inputs=2
  Mux3 : Mux  Inputs=3
  Phi : Scope
  Posición : Scope
  Psi : Scope
  Radians to Degrees{1..7} (7 alike) : simulink_extras/Transformations/Radians to Degrees
  Terminator3 : Terminator
  Terminator4 : Terminator
  Theta : Scope
  Theta1 : Scope
  To Workspace : ToWorkspace  VariableName=Theta1  SampleTime=-1
  To Workspace1 : ToWorkspace  VariableName=Phi1  SampleTime=-1
  To Workspace2 : ToWorkspace  VariableName=Psi1  SampleTime=-1
  To Workspace3 : ToWorkspace  VariableName=Height1  SampleTime=-1
  To Workspace4 : ToWorkspace  VariableName=Beta1  SampleTime=-1
  To Workspace5 : ToWorkspace  VariableName=Speed1  SampleTime=-1
  To Workspace6 : ToWorkspace  VariableName=Alpha1  SampleTime=-1
  To Workspace7 : ToWorkspace  VariableName=Gamma1  SampleTime=-1
  To Workspace8 : ToWorkspace  VariableName=Position_x1  SampleTime=-1
  To Workspace9 : ToWorkspace  VariableName=Position_y1  SampleTime=-1
  "Velocidad ejes tierra " : Scope
  position_x : Scope
  position_y : Scope
  theta-alpha=gamma : Sum  Inputs=+-
  Lwb1 : Outport
  Lbw1 : Outport  Port=2
  "Lbw " : Outport  Port=3
  Lwb : Outport  Port=4
  X_e : Outport  Port=5
  "Navigation angles " : Outport  Port=6
  Phi[deg] : Outport  Port=7
  Theta[deg] : Outport  Port=8
  Psi[deg] : Outport  Port=9
  theta : Outport  Port=10
  beta : Outport  Port=11
  alpha : Outport  Port=12
  V : Outport  Port=13
  theta' : Outport  Port=14
  h : Outport  Port=15
  gamma : Outport  Port=16
  wires:
  Direction Cosine Matrix Body to Wind/1 -> Lwb/1, Invert 3x3 Matrix/1
  Radians to Degrees3/1 -> To Workspace6/1
  theta-alpha=gamma/1 -> gamma/1, Radians to Degrees4/1
  Invert 3x3 Matrix/1 -> "Lbw "/1
  Mux1/1 -> Direction Cosine Matrix Body to Wind1/1
  Demux3/3 -> Gain/1, h/1, To Workspace3/1
  V_e/1 -> "Velocidad ejes tierra "/1
  omega/1 -> Demux1/1
  "Incidence, Sideslip, & Airspeed"/2 -> beta/1, Radians to Degrees7/1, Mux2/2, Mux1/2
  V_b/1 -> "Incidence, Sideslip, & Airspeed"/1
  x_e/1 -> Demux3/1, Posición/1
  Mux2/1 -> Direction Cosine Matrix Body to Wind/1
  Direction Cosine Matrix Body to Wind1/1 -> Lwb1/1, Invert 3x3 Matrix1/1
  "Incidence, Sideslip, & Airspeed"/1 -> Mux2/1, alpha/1, Radians to Degrees3/1, theta-alpha=gamma/2
  Radians to Degrees2/1 -> To Workspace/1, Theta1/1, Theta[deg]/1
  Demux1/3 -> Terminator4/1
  Demux1/2 -> theta'/1
  Invert 3x3 Matrix1/1 -> Lbw1/1
  Demux1/1 -> Terminator3/1
  Demux2/1 -> Radians to Degrees6/1
  Demux3/2 -> position_y/1, Mux3/2, To Workspace9/1
  Radians to Degrees1/1 -> Angles/1
  Demux3/1 -> Mux3/1, position_x/1, To Workspace8/1
  Demux2/2 -> theta-alpha=gamma/1, Theta/1, theta/1, Mux1/1, Radians to Degrees2/1
  Radians to Degrees4/1 -> To Workspace7/1
  "Incidence, Sideslip, & Airspeed"/3 -> V/1, To Workspace5/1
  Demux2/3 -> Radians to Degrees5/1
  Radians to Degrees5/1 -> To Workspace2/1, Psi/1, Psi[deg]/1
  Radians to Degrees6/1 -> To Workspace1/1, Phi/1, Phi[deg]/1
  Radians to Degrees7/1 -> To Workspace4/1
  Mux3/1 -> X_e/1
  Gain/1 -> Altura/1, Mux3/3
  Navigation angles/1 -> "Navigation angles "/1, Radians to Degrees1/1, Demux2/1

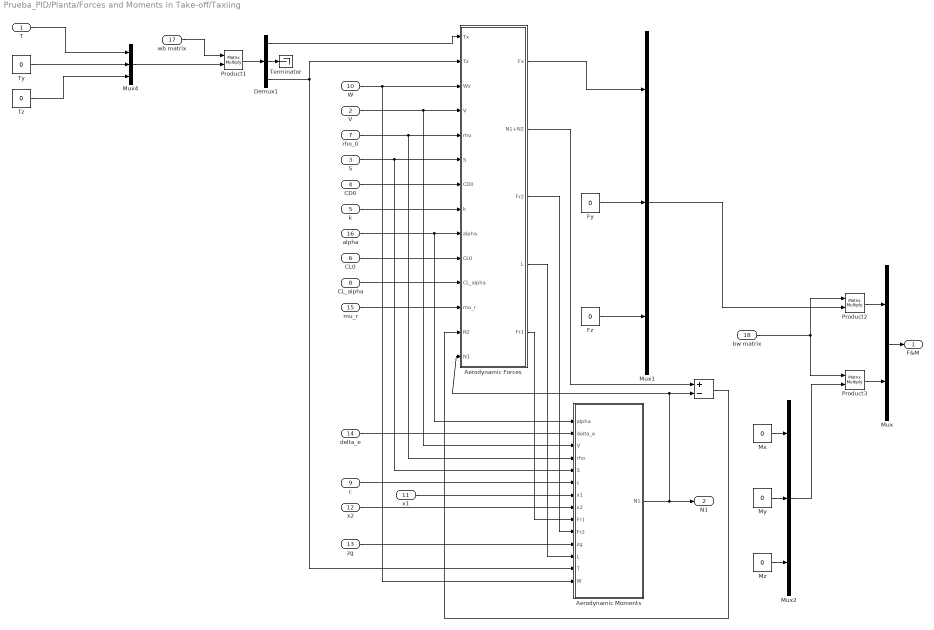
== system Prueba_PID/Planta/Forces and Moments in Take-off/Taxiing ==
  T : Inport
  V : Inport  Port=2
  S : Inport  Port=3
  CD0 : Inport  Port=4
  k : Inport  Port=5
  CL0 : Inport  Port=6
  rho_0 : Inport  Port=7
  CL_alpha : Inport  Port=8
  c : Inport  Port=9
  W : Inport  Port=10
  x1 : Inport  Port=11
  x2 : Inport  Port=12
  zg : Inport  Port=13
  delta_e : Inport  Port=14
  mu_r : Inport  Port=15
  alpha : Inport  Port=16
  wb matrix : Inport  Port=17
  bw matrix : Inport  Port=18
  " " : Sum  Inputs=+-
  "Aerodynamic Forces " : Subsystem
  "Aerodynamic Moments " : Subsystem
  Demux1 : Demux  Outputs=3
  Fy : Constant  Value=0
  Fz : Constant  Value=0
  Mux : Mux  Inputs=2
  Mux1 : Mux  Inputs=3
  Mux2 : Mux  Inputs=3
  Mux4 : Mux  Inputs=3
  Mx : Constant  Value=0
  My : Constant  Value=0
  Mz : Constant  Value=0
  Product1 : Product  Multiplication=Matrix(*)
  Product2 : Product  Multiplication=Matrix(*)
  Product3 : Product  Multiplication=Matrix(*)
  Terminator : Terminator
  Ty : Constant  Value=0
  Tz : Constant  Value=0
  F&M : Outport
  N1 : Outport  Port=2
  wires:
  Mux/1 -> F&M/1
  T/1 -> Mux4/1
  Ty/1 -> Mux4/2
  Tz/1 -> Mux4/3
  Mux4/1 -> Product1/2
  Product1/1 -> Demux1/1
  Demux1/2 -> Terminator/1
  wb matrix/1 -> Product1/1
  Mux1/1 -> Product2/2
  bw matrix/1 -> Product2/1, Product3/1
  Product2/1 -> Mux/1
  Product3/1 -> Mux/2
  Mux2/1 -> Product3/2
  "Aerodynamic Forces "/1(Fx) -> Mux1/1
  Demux1/1 -> "Aerodynamic Forces "/1("Tx ")
  alpha/1 -> "Aerodynamic Forces "/9(alpha), "Aerodynamic Moments "/1(alpha)
  Demux1/3 -> "Aerodynamic Moments "/13(T), "Aerodynamic Forces "/2("Tz ")
  c/1 -> "Aerodynamic Moments "/6(c)
  delta_e/1 -> "Aerodynamic Moments "/2(delta_e)
  W/1 -> "Aerodynamic Moments "/14(W), "Aerodynamic Forces "/3(Wz)
  V/1 -> "Aerodynamic Moments "/3(V), "Aerodynamic Forces "/4(V)
  S/1 -> "Aerodynamic Moments "/5(S), "Aerodynamic Forces "/6(S)
  CD0/1 -> "Aerodynamic Forces "/7(CD0)
  k/1 -> "Aerodynamic Forces "/8(k)
  CL_alpha/1 -> "Aerodynamic Forces "/11(CL_alpha)
  CL0/1 -> "Aerodynamic Forces "/10(CL0)
  rho_0/1 -> "Aerodynamic Moments "/4(rho), "Aerodynamic Forces "/5(rho)
  Fy/1 -> Mux1/2
  Fz/1 -> Mux1/3
  mu_r/1 -> "Aerodynamic Forces "/12(mu_r)
  Mx/1 -> Mux2/1
  Mz/1 -> Mux2/3
  x2/1 -> "Aerodynamic Moments "/8(x2)
  zg/1 -> "Aerodynamic Moments "/11(zg)
  "Aerodynamic Forces "/3(Fr2) -> "Aerodynamic Moments "/10(Fr2)
  My/1 -> Mux2/2
  "Aerodynamic Forces "/2(N1+N2) -> " "/1
  " "/1 -> "Aerodynamic Forces "/13(N2)
  "Aerodynamic Moments "/1(N1) -> N1/1, "Aerodynamic Forces "/14(N1), " "/2
  "Aerodynamic Forces "/4(L) -> "Aerodynamic Moments "/12(L)
  "Aerodynamic Forces "/5(Fr1) -> "Aerodynamic Moments "/9(Fr1)
  x1/1 -> "Aerodynamic Moments "/7(x1)

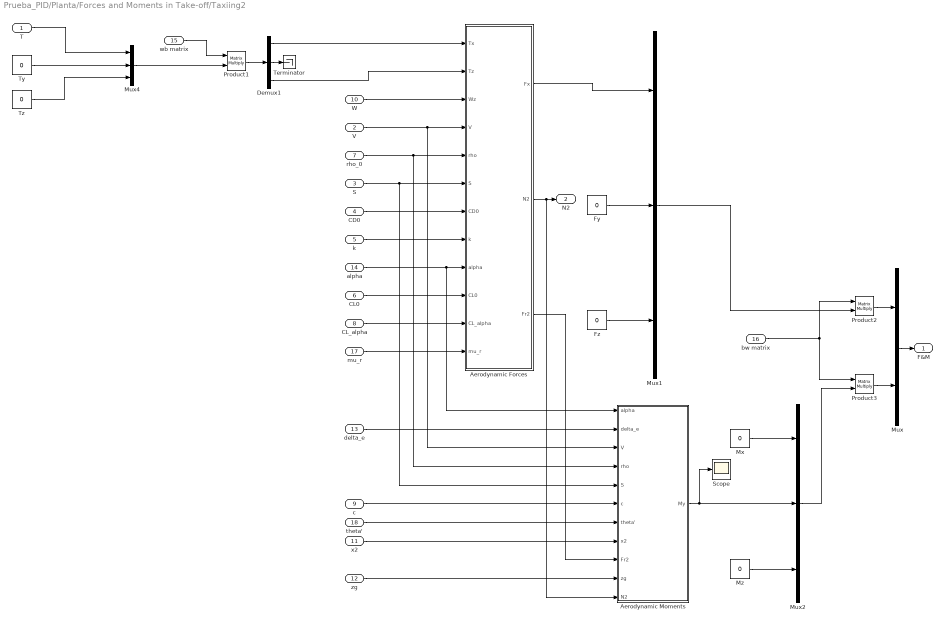
== system Prueba_PID/Planta/Forces and Moments in Take-off/Taxiing2 ==
  T : Inport
  V : Inport  Port=2
  S : Inport  Port=3
  CD0 : Inport  Port=4
  k : Inport  Port=5
  CL0 : Inport  Port=6
  rho_0 : Inport  Port=7
  CL_alpha : Inport  Port=8
  c : Inport  Port=9
  W : Inport  Port=10
  x2 : Inport  Port=11
  zg : Inport  Port=12
  delta_e : Inport  Port=13
  alpha : Inport  Port=14
  wb matrix : Inport  Port=15
  bw matrix : Inport  Port=16
  mu_r : Inport  Port=17
  theta' : Inport  Port=18
  "Aerodynamic Forces " : Subsystem
  "Aerodynamic Moments " : Subsystem
  Demux1 : Demux  Outputs=3
  Fy : Constant  Value=0
  Fz : Constant  Value=0
  Mux : Mux  Inputs=2
  Mux1 : Mux  Inputs=3
  Mux2 : Mux  Inputs=3
  Mux4 : Mux  Inputs=3
  Mx : Constant  Value=0
  Mz : Constant  Value=0
  Product1 : Product  Multiplication=Matrix(*)
  Product2 : Product  Multiplication=Matrix(*)
  Product3 : Product  Multiplication=Matrix(*)
  Scope : Scope
  Terminator : Terminator
  Ty : Constant  Value=0
  Tz : Constant  Value=0
  F&M : Outport
  N2 : Outport  Port=2
  wires:
  Mux/1 -> F&M/1
  T/1 -> Mux4/1
  Ty/1 -> Mux4/2
  Tz/1 -> Mux4/3
  Mux4/1 -> Product1/2
  Product1/1 -> Demux1/1
  Demux1/2 -> Terminator/1
  wb matrix/1 -> Product1/1
  Mux1/1 -> Product2/2
  bw matrix/1 -> Product2/1, Product3/1
  Product2/1 -> Mux/1
  Product3/1 -> Mux/2
  Mux2/1 -> Product3/2
  "Aerodynamic Forces "/1(Fx) -> Mux1/1
  "Aerodynamic Moments "/1(My) -> Scope/1, Mux2/2
  Demux1/1 -> "Aerodynamic Forces "/1("Tx ")
  alpha/1 -> "Aerodynamic Moments "/1(alpha), "Aerodynamic Forces "/9(alpha)
  Demux1/3 -> "Aerodynamic Forces "/2("Tz ")
  c/1 -> "Aerodynamic Moments "/6(c)
  delta_e/1 -> "Aerodynamic Moments "/2(delta_e)
  W/1 -> "Aerodynamic Forces "/3(Wz)
  V/1 -> "Aerodynamic Moments "/3(V), "Aerodynamic Forces "/4(V)
  S/1 -> "Aerodynamic Moments "/5(S), "Aerodynamic Forces "/6(S)
  CD0/1 -> "Aerodynamic Forces "/7(CD0)
  k/1 -> "Aerodynamic Forces "/8(k)
  CL_alpha/1 -> "Aerodynamic Forces "/11(CL_alpha)
  CL0/1 -> "Aerodynamic Forces "/10(CL0)
  rho_0/1 -> "Aerodynamic Moments "/4(rho), "Aerodynamic Forces "/5(rho)
  Fy/1 -> Mux1/2
  Fz/1 -> Mux1/3
  "Aerodynamic Forces "/2(N2) -> "Aerodynamic Moments "/11(N2), N2/1
  mu_r/1 -> "Aerodynamic Forces "/12(mu_r)
  theta'/1 -> "Aerodynamic Moments "/7(theta')
  Mx/1 -> Mux2/1
  Mz/1 -> Mux2/3
  x2/1 -> "Aerodynamic Moments "/8(x2)
  zg/1 -> "Aerodynamic Moments "/10(zg)
  "Aerodynamic Forces "/3(Fr2) -> "Aerodynamic Moments "/9(Fr2)

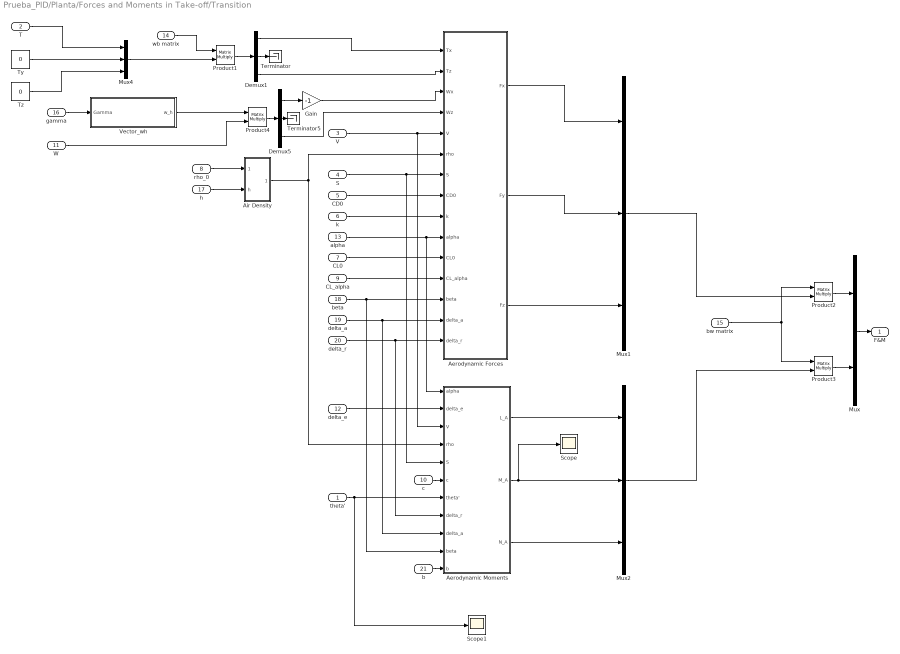
== system Prueba_PID/Planta/Forces and Moments in Take-off/Transition ==
  theta' : Inport
  T : Inport  Port=2
  V : Inport  Port=3
  S : Inport  Port=4
  CD0 : Inport  Port=5
  k : Inport  Port=6
  CL0 : Inport  Port=7
  rho_0 : Inport  Port=8
  CL_alpha : Inport  Port=9
  c : Inport  Port=10
  W : Inport  Port=11
  delta_e : Inport  Port=12
  alpha : Inport  Port=13
  wb matrix : Inport  Port=14
  bw matrix : Inport  Port=15
  gamma : Inport  Port=16
  h : Inport  Port=17
  beta : Inport  Port=18
  delta_a : Inport  Port=19
  delta_r : Inport  Port=20
  b : Inport  Port=21
  "Aerodynamic Forces " : Subsystem
  "Aerodynamic Moments " : Subsystem
  Air Density : Subsystem
  Demux1 : Demux  Outputs=3
  Demux5 : Demux  Outputs=3
  Gain : Gain  Gain=-1
  Mux : Mux  Inputs=2
  Mux1 : Mux  Inputs=3
  Mux2 : Mux  Inputs=3
  Mux4 : Mux  Inputs=3
  Product{1..4} (4 alike) : Product  Multiplication=Matrix(*)
  Scope : Scope
  Scope1 : Scope
  Terminator : Terminator
  Terminator5 : Terminator
  Ty : Constant  Value=0
  Tz : Constant  Value=0
  Vector_wh : Subsystem
  F&M : Outport
  wires:
  Mux/1 -> F&M/1
  T/1 -> Mux4/1
  Ty/1 -> Mux4/2
  Tz/1 -> Mux4/3
  Mux4/1 -> Product1/2
  Product1/1 -> Demux1/1
  Demux1/2 -> Terminator/1
  wb matrix/1 -> Product1/1
  Mux1/1 -> Product2/2
  bw matrix/1 -> Product2/1, Product3/1
  Product2/1 -> Mux/1
  Product3/1 -> Mux/2
  Mux2/1 -> Product3/2
  gamma/1 -> Vector_wh/1(Gamma)
  Demux5/2 -> Terminator5/1
  Product4/1 -> Demux5/1
  W/1 -> Product4/2
  Vector_wh/1(w_h) -> Product4/1
  Demux5/1 -> Gain/1
  rho_0/1 -> Air Density/1(rho_0)
  h/1 -> Air Density/2(h)
  "Aerodynamic Forces "/1(Fx) -> Mux1/1
  "Aerodynamic Forces "/2(Fy) -> Mux1/2
  "Aerodynamic Forces "/3(Fz) -> Mux1/3
  "Aerodynamic Moments "/1("L_A ") -> Mux2/1
  "Aerodynamic Moments "/2(M_A) -> Scope/1, Mux2/2
  "Aerodynamic Moments "/3(N_A) -> Mux2/3
  Demux1/1 -> "Aerodynamic Forces "/1("Tx ")
  alpha/1 -> "Aerodynamic Moments "/1(alpha), "Aerodynamic Forces "/10(alpha)
  Demux1/3 -> "Aerodynamic Forces "/2("Tz ")
  c/1 -> "Aerodynamic Moments "/6(c)
  delta_e/1 -> "Aerodynamic Moments "/2(delta_e)
  theta'/1 -> "Aerodynamic Moments "/7(theta'), Scope1/1
  Gain/1 -> "Aerodynamic Forces "/3(Wx)
  Demux5/3 -> "Aerodynamic Forces "/4(Wz)
  V/1 -> "Aerodynamic Moments "/3(V), "Aerodynamic Forces "/5(V)
  S/1 -> "Aerodynamic Forces "/7(S), "Aerodynamic Moments "/5(S)
  CD0/1 -> "Aerodynamic Forces "/8(CD0)
  k/1 -> "Aerodynamic Forces "/9(k)
  CL_alpha/1 -> "Aerodynamic Forces "/12(CL_alpha)
  CL0/1 -> "Aerodynamic Forces "/11(CL0)
  Air Density/1("rho ") -> "Aerodynamic Moments "/4(rho), "Aerodynamic Forces "/6(rho)
  beta/1 -> "Aerodynamic Forces "/13(beta), "Aerodynamic Moments "/10(beta)
  delta_a/1 -> "Aerodynamic Forces "/14(delta_a), "Aerodynamic Moments "/9(delta_a)
  delta_r/1 -> "Aerodynamic Forces "/15(delta_r), "Aerodynamic Moments "/8(delta_r)
  b/1 -> "Aerodynamic Moments "/11(b)

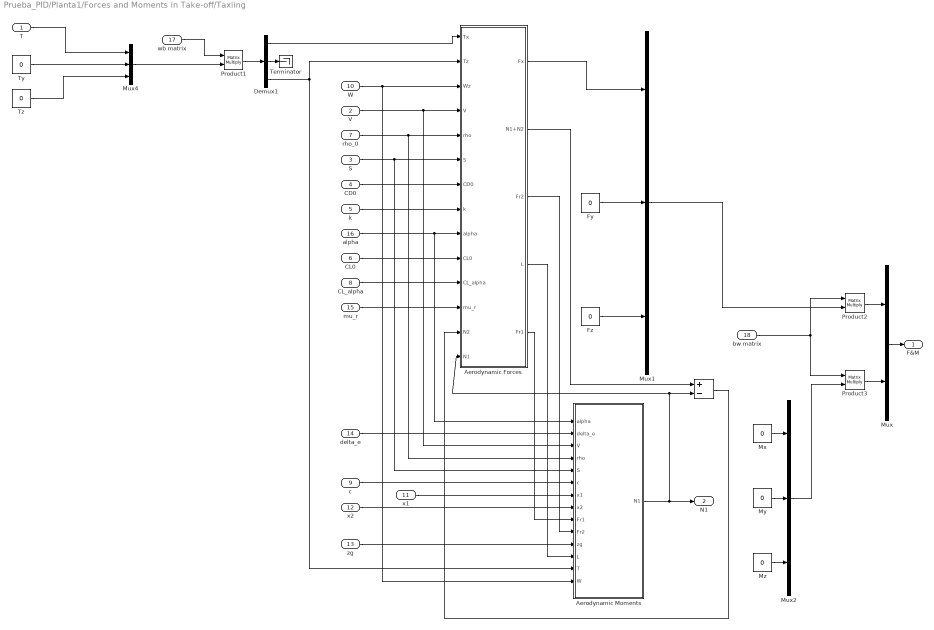
== system Prueba_PID/Planta1/Forces and Moments in Take-off/Taxiing ==
  T : Inport
  V : Inport  Port=2
  S : Inport  Port=3
  CD0 : Inport  Port=4
  k : Inport  Port=5
  CL0 : Inport  Port=6
  rho_0 : Inport  Port=7
  CL_alpha : Inport  Port=8
  c : Inport  Port=9
  W : Inport  Port=10
  x1 : Inport  Port=11
  x2 : Inport  Port=12
  zg : Inport  Port=13
  delta_e : Inport  Port=14
  mu_r : Inport  Port=15
  alpha : Inport  Port=16
  wb matrix : Inport  Port=17
  bw matrix : Inport  Port=18
  " " : Sum  Inputs=+-
  "Aerodynamic Forces " : Subsystem
  "Aerodynamic Moments " : Subsystem
  Demux1 : Demux  Outputs=3
  Fy : Constant  Value=0
  Fz : Constant  Value=0
  Mux : Mux  Inputs=2
  Mux1 : Mux  Inputs=3
  Mux2 : Mux  Inputs=3
  Mux4 : Mux  Inputs=3
  Mx : Constant  Value=0
  My : Constant  Value=0
  Mz : Constant  Value=0
  Product1 : Product  Multiplication=Matrix(*)
  Product2 : Product  Multiplication=Matrix(*)
  Product3 : Product  Multiplication=Matrix(*)
  Terminator : Terminator
  Ty : Constant  Value=0
  Tz : Constant  Value=0
  F&M : Outport
  N1 : Outport  Port=2
  wires:
  Mux/1 -> F&M/1
  T/1 -> Mux4/1
  Ty/1 -> Mux4/2
  Tz/1 -> Mux4/3
  Mux4/1 -> Product1/2
  Product1/1 -> Demux1/1
  Demux1/2 -> Terminator/1
  wb matrix/1 -> Product1/1
  Mux1/1 -> Product2/2
  bw matrix/1 -> Product2/1, Product3/1
  Product2/1 -> Mux/1
  Product3/1 -> Mux/2
  Mux2/1 -> Product3/2
  "Aerodynamic Forces "/1(Fx) -> Mux1/1
  Demux1/1 -> "Aerodynamic Forces "/1("Tx ")
  alpha/1 -> "Aerodynamic Forces "/9(alpha), "Aerodynamic Moments "/1(alpha)
  Demux1/3 -> "Aerodynamic Moments "/13(T), "Aerodynamic Forces "/2("Tz ")
  c/1 -> "Aerodynamic Moments "/6(c)
  delta_e/1 -> "Aerodynamic Moments "/2(delta_e)
  W/1 -> "Aerodynamic Moments "/14(W), "Aerodynamic Forces "/3(Wz)
  V/1 -> "Aerodynamic Moments "/3(V), "Aerodynamic Forces "/4(V)
  S/1 -> "Aerodynamic Moments "/5(S), "Aerodynamic Forces "/6(S)
  CD0/1 -> "Aerodynamic Forces "/7(CD0)
  k/1 -> "Aerodynamic Forces "/8(k)
  CL_alpha/1 -> "Aerodynamic Forces "/11(CL_alpha)
  CL0/1 -> "Aerodynamic Forces "/10(CL0)
  rho_0/1 -> "Aerodynamic Moments "/4(rho), "Aerodynamic Forces "/5(rho)
  Fy/1 -> Mux1/2
  Fz/1 -> Mux1/3
  mu_r/1 -> "Aerodynamic Forces "/12(mu_r)
  Mx/1 -> Mux2/1
  Mz/1 -> Mux2/3
  x2/1 -> "Aerodynamic Moments "/8(x2)
  zg/1 -> "Aerodynamic Moments "/11(zg)
  "Aerodynamic Forces "/3(Fr2) -> "Aerodynamic Moments "/10(Fr2)
  My/1 -> Mux2/2
  "Aerodynamic Forces "/2(N1+N2) -> " "/1
  " "/1 -> "Aerodynamic Forces "/13(N2)
  "Aerodynamic Moments "/1(N1) -> N1/1, "Aerodynamic Forces "/14(N1), " "/2
  "Aerodynamic Forces "/4(L) -> "Aerodynamic Moments "/12(L)
  "Aerodynamic Forces "/5(Fr1) -> "Aerodynamic Moments "/9(Fr1)
  x1/1 -> "Aerodynamic Moments "/7(x1)

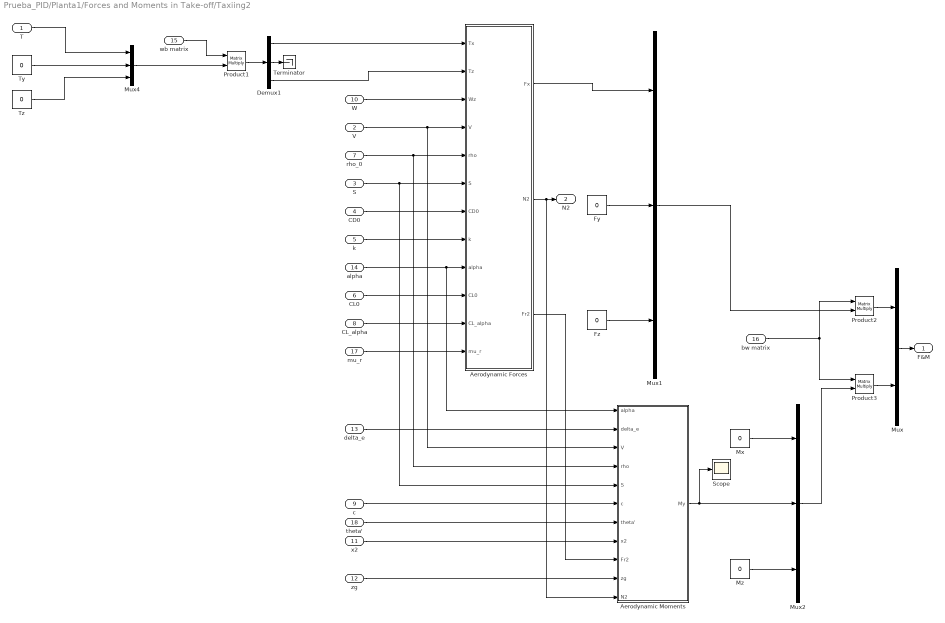
== system Prueba_PID/Planta1/Forces and Moments in Take-off/Taxiing2 ==
  T : Inport
  V : Inport  Port=2
  S : Inport  Port=3
  CD0 : Inport  Port=4
  k : Inport  Port=5
  CL0 : Inport  Port=6
  rho_0 : Inport  Port=7
  CL_alpha : Inport  Port=8
  c : Inport  Port=9
  W : Inport  Port=10
  x2 : Inport  Port=11
  zg : Inport  Port=12
  delta_e : Inport  Port=13
  alpha : Inport  Port=14
  wb matrix : Inport  Port=15
  bw matrix : Inport  Port=16
  mu_r : Inport  Port=17
  theta' : Inport  Port=18
  "Aerodynamic Forces " : Subsystem
  "Aerodynamic Moments " : Subsystem
  Demux1 : Demux  Outputs=3
  Fy : Constant  Value=0
  Fz : Constant  Value=0
  Mux : Mux  Inputs=2
  Mux1 : Mux  Inputs=3
  Mux2 : Mux  Inputs=3
  Mux4 : Mux  Inputs=3
  Mx : Constant  Value=0
  Mz : Constant  Value=0
  Product1 : Product  Multiplication=Matrix(*)
  Product2 : Product  Multiplication=Matrix(*)
  Product3 : Product  Multiplication=Matrix(*)
  Scope : Scope
  Terminator : Terminator
  Ty : Constant  Value=0
  Tz : Constant  Value=0
  F&M : Outport
  N2 : Outport  Port=2
  wires:
  Mux/1 -> F&M/1
  T/1 -> Mux4/1
  Ty/1 -> Mux4/2
  Tz/1 -> Mux4/3
  Mux4/1 -> Product1/2
  Product1/1 -> Demux1/1
  Demux1/2 -> Terminator/1
  wb matrix/1 -> Product1/1
  Mux1/1 -> Product2/2
  bw matrix/1 -> Product2/1, Product3/1
  Product2/1 -> Mux/1
  Product3/1 -> Mux/2
  Mux2/1 -> Product3/2
  "Aerodynamic Forces "/1(Fx) -> Mux1/1
  "Aerodynamic Moments "/1(My) -> Scope/1, Mux2/2
  Demux1/1 -> "Aerodynamic Forces "/1("Tx ")
  alpha/1 -> "Aerodynamic Moments "/1(alpha), "Aerodynamic Forces "/9(alpha)
  Demux1/3 -> "Aerodynamic Forces "/2("Tz ")
  c/1 -> "Aerodynamic Moments "/6(c)
  delta_e/1 -> "Aerodynamic Moments "/2(delta_e)
  W/1 -> "Aerodynamic Forces "/3(Wz)
  V/1 -> "Aerodynamic Moments "/3(V), "Aerodynamic Forces "/4(V)
  S/1 -> "Aerodynamic Moments "/5(S), "Aerodynamic Forces "/6(S)
  CD0/1 -> "Aerodynamic Forces "/7(CD0)
  k/1 -> "Aerodynamic Forces "/8(k)
  CL_alpha/1 -> "Aerodynamic Forces "/11(CL_alpha)
  CL0/1 -> "Aerodynamic Forces "/10(CL0)
  rho_0/1 -> "Aerodynamic Moments "/4(rho), "Aerodynamic Forces "/5(rho)
  Fy/1 -> Mux1/2
  Fz/1 -> Mux1/3
  "Aerodynamic Forces "/2(N2) -> "Aerodynamic Moments "/11(N2), N2/1
  mu_r/1 -> "Aerodynamic Forces "/12(mu_r)
  theta'/1 -> "Aerodynamic Moments "/7(theta')
  Mx/1 -> Mux2/1
  Mz/1 -> Mux2/3
  x2/1 -> "Aerodynamic Moments "/8(x2)
  zg/1 -> "Aerodynamic Moments "/10(zg)
  "Aerodynamic Forces "/3(Fr2) -> "Aerodynamic Moments "/9(Fr2)

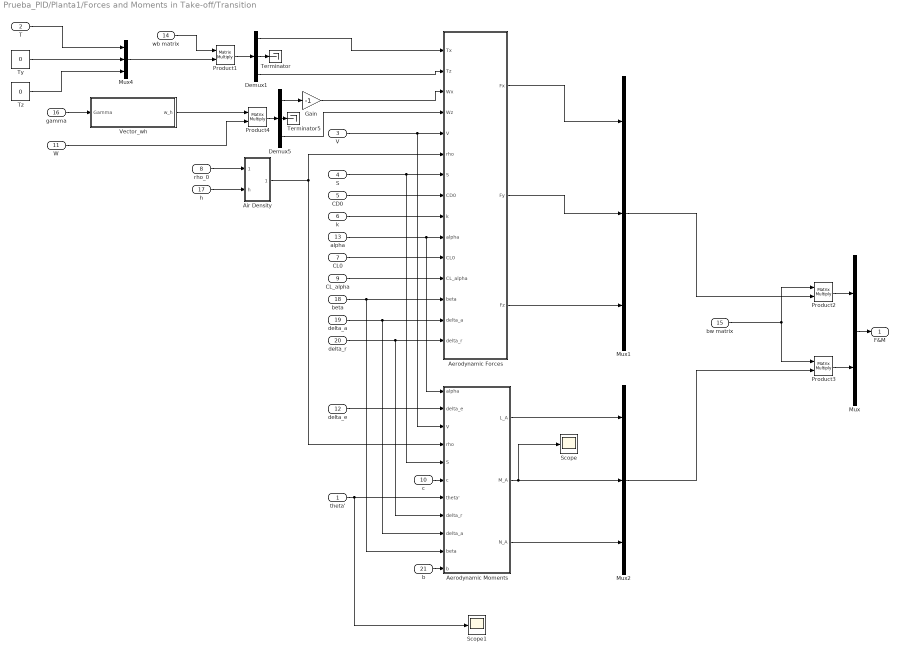
== system Prueba_PID/Planta1/Forces and Moments in Take-off/Transition ==
  theta' : Inport
  T : Inport  Port=2
  V : Inport  Port=3
  S : Inport  Port=4
  CD0 : Inport  Port=5
  k : Inport  Port=6
  CL0 : Inport  Port=7
  rho_0 : Inport  Port=8
  CL_alpha : Inport  Port=9
  c : Inport  Port=10
  W : Inport  Port=11
  delta_e : Inport  Port=12
  alpha : Inport  Port=13
  wb matrix : Inport  Port=14
  bw matrix : Inport  Port=15
  gamma : Inport  Port=16
  h : Inport  Port=17
  beta : Inport  Port=18
  delta_a : Inport  Port=19
  delta_r : Inport  Port=20
  b : Inport  Port=21
  "Aerodynamic Forces " : Subsystem
  "Aerodynamic Moments " : Subsystem
  Air Density : Subsystem
  Demux1 : Demux  Outputs=3
  Demux5 : Demux  Outputs=3
  Gain : Gain  Gain=-1
  Mux : Mux  Inputs=2
  Mux1 : Mux  Inputs=3
  Mux2 : Mux  Inputs=3
  Mux4 : Mux  Inputs=3
  Product{1..4} (4 alike) : Product  Multiplication=Matrix(*)
  Scope : Scope
  Scope1 : Scope
  Terminator : Terminator
  Terminator5 : Terminator
  Ty : Constant  Value=0
  Tz : Constant  Value=0
  Vector_wh : Subsystem
  F&M : Outport
  wires:
  Mux/1 -> F&M/1
  T/1 -> Mux4/1
  Ty/1 -> Mux4/2
  Tz/1 -> Mux4/3
  Mux4/1 -> Product1/2
  Product1/1 -> Demux1/1
  Demux1/2 -> Terminator/1
  wb matrix/1 -> Product1/1
  Mux1/1 -> Product2/2
  bw matrix/1 -> Product2/1, Product3/1
  Product2/1 -> Mux/1
  Product3/1 -> Mux/2
  Mux2/1 -> Product3/2
  gamma/1 -> Vector_wh/1(Gamma)
  Demux5/2 -> Terminator5/1
  Product4/1 -> Demux5/1
  W/1 -> Product4/2
  Vector_wh/1(w_h) -> Product4/1
  Demux5/1 -> Gain/1
  rho_0/1 -> Air Density/1(rho_0)
  h/1 -> Air Density/2(h)
  "Aerodynamic Forces "/1(Fx) -> Mux1/1
  "Aerodynamic Forces "/2(Fy) -> Mux1/2
  "Aerodynamic Forces "/3(Fz) -> Mux1/3
  "Aerodynamic Moments "/1("L_A ") -> Mux2/1
  "Aerodynamic Moments "/2(M_A) -> Scope/1, Mux2/2
  "Aerodynamic Moments "/3(N_A) -> Mux2/3
  Demux1/1 -> "Aerodynamic Forces "/1("Tx ")
  alpha/1 -> "Aerodynamic Moments "/1(alpha), "Aerodynamic Forces "/10(alpha)
  Demux1/3 -> "Aerodynamic Forces "/2("Tz ")
  c/1 -> "Aerodynamic Moments "/6(c)
  delta_e/1 -> "Aerodynamic Moments "/2(delta_e)
  theta'/1 -> "Aerodynamic Moments "/7(theta'), Scope1/1
  Gain/1 -> "Aerodynamic Forces "/3(Wx)
  Demux5/3 -> "Aerodynamic Forces "/4(Wz)
  V/1 -> "Aerodynamic Moments "/3(V), "Aerodynamic Forces "/5(V)
  S/1 -> "Aerodynamic Forces "/7(S), "Aerodynamic Moments "/5(S)
  CD0/1 -> "Aerodynamic Forces "/8(CD0)
  k/1 -> "Aerodynamic Forces "/9(k)
  CL_alpha/1 -> "Aerodynamic Forces "/12(CL_alpha)
  CL0/1 -> "Aerodynamic Forces "/11(CL0)
  Air Density/1("rho ") -> "Aerodynamic Moments "/4(rho), "Aerodynamic Forces "/6(rho)
  beta/1 -> "Aerodynamic Forces "/13(beta), "Aerodynamic Moments "/10(beta)
  delta_a/1 -> "Aerodynamic Forces "/14(delta_a), "Aerodynamic Moments "/9(delta_a)
  delta_r/1 -> "Aerodynamic Forces "/15(delta_r), "Aerodynamic Moments "/8(delta_r)
  b/1 -> "Aerodynamic Moments "/11(b)
